simulink model "present1"  (Simulink 7.6)
settings: Solver=ode45  StartTime=0.0  StopTime=10.0  RelTol=1e-3
settings Model: Creator=jordan  LastModifiedBy=jordan

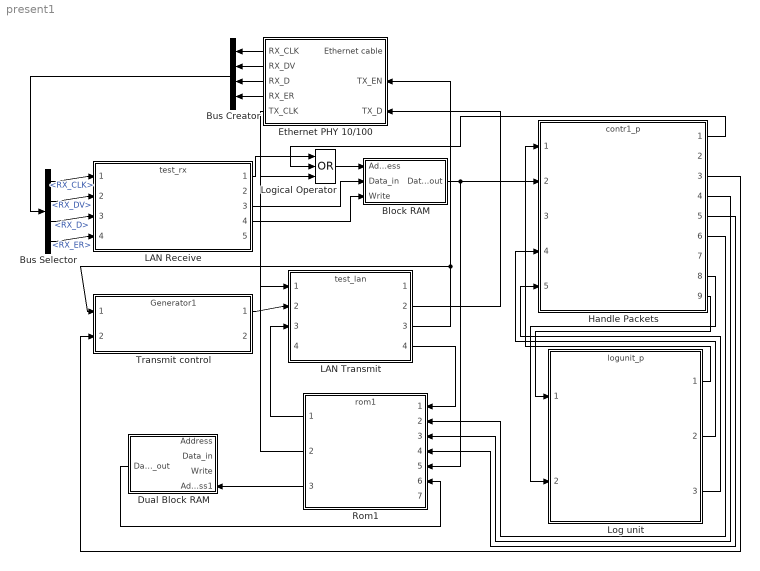
== system present1 ==
  Block RAM : Subsystem
  Bus Creator : BusCreator  Inputs='RX_CLK','RX_DV','RX_D','RX_ER'
  Bus Selector : BusSelector  OutputSignals=RX_CLK,RX_DV,RX_D,RX_ER
  Dual Block RAM : Subsystem
  Ethernet PHY 10/100 : Subsystem
  Handle Packets : ModelReference  ModelNameDialog=contr1_p  SimulationMode=Normal  ModelReferenceVersion=1.463  CopyOfModelName=contr1_p
  LAN Receive : ModelReference  ModelNameDialog=test_rx  SimulationMode=Normal  ModelReferenceVersion=1.280  CopyOfModelName=test_rx
  LAN Transmit : ModelReference  ModelNameDialog=test_lan  SimulationMode=Normal  ModelReferenceVersion=1.197  CopyOfModelName=test_lan
  Log unit : ModelReference  ModelNameDialog=logunit_p  SimulationMode=Normal  ModelReferenceVersion=1.518  CopyOfModelName=logunit_p
  Logical Operator : Logic  Operator=OR  Inputs=3  AllPortsSameDT=off  OutDataTypeStr=boolean
  Rom1 : ModelReference  ModelNameDialog=rom1  SimulationMode=Normal  ModelReferenceVersion=1.162  CopyOfModelName=rom1
  Transmit control : ModelReference  ModelNameDialog=Generator1  SimulationMode=Normal  ModelReferenceVersion=1.103  CopyOfModelName=Generator1
  wires:
  Block RAM/1(Data_out) -> Handle Packets/2, Rom1/5
  LAN Receive/3 -> Block RAM/2(Data_in)
  LAN Receive/4 -> Block RAM/3(Write)
  LAN Receive/1 -> Logical Operator/1
  Transmit control/1 -> LAN Transmit/2
  LAN Transmit/3 -> Transmit control/1, Ethernet PHY 10/100/2(TX_EN)
  Logical Operator/1 -> Block RAM/1(Address)
  Rom1/1 -> LAN Transmit/3
  LAN Transmit/4 -> Rom1/1
  Rom1/2 -> Logical Operator/3
  Ethernet PHY 10/100/1(RX_CLK) -> Bus Creator/1
  Ethernet PHY 10/100/2(RX_DV) -> Bus Creator/2
  Ethernet PHY 10/100/3(RX_D) -> Bus Creator/3
  Ethernet PHY 10/100/4(RX_ER) -> Bus Creator/4
  Bus Selector/1 -> LAN Receive/1  "<RX_CLK>"
  Bus Selector/2 -> LAN Receive/2  "<RX_DV>"
  Bus Selector/3 -> LAN Receive/3  "<RX_D>"
  Bus Selector/4 -> LAN Receive/4  "<RX_ER>"
  LAN Transmit/2 -> Ethernet PHY 10/100/3(TX_D)
  Ethernet PHY 10/100/5(TX_CLK) -> LAN Transmit/1
  Dual Block RAM/1(Data_out) -> Rom1/6
  Rom1/3 -> Dual Block RAM/4(Address1)
  Log unit/1 -> Handle Packets/1
  Bus Creator/1 -> Bus Selector/1
  Log unit/2 -> Handle Packets/4
  Log unit/3 -> Handle Packets/5
  Handle Packets/1 -> Logical Operator/2
  Handle Packets/6 -> Rom1/2
  Handle Packets/4 -> Rom1/3
  Handle Packets/5 -> Rom1/4
  Handle Packets/3 -> Transmit control/2
  Handle Packets/9 -> Log unit/1
  Handle Packets/8 -> Log unit/2

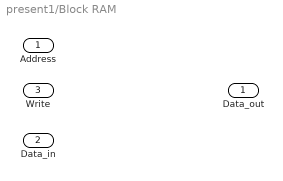
== system present1/Block RAM ==
  Address : Inport  OutDataTypeStr=boolean
  Data_in : Inport  Port=2  OutDataTypeStr=boolean
  Write : Inport  Port=3  OutDataTypeStr=boolean
  Data_out : Outport

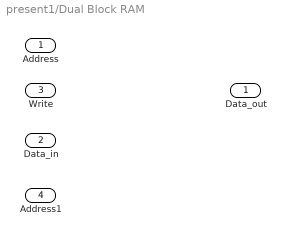
== system present1/Dual Block RAM ==
  Address : Inport  OutDataTypeStr=boolean
  Data_in : Inport  Port=2  OutDataTypeStr=boolean
  Write : Inport  Port=3  OutDataTypeStr=boolean
  Address1 : Inport  Port=4  OutDataTypeStr=boolean
  Data_out : Outport

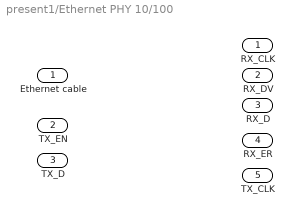
== system present1/Ethernet PHY 10/100 ==
  Ethernet cable : Inport  OutDataTypeStr=boolean
  TX_EN : Inport  Port=2  OutDataTypeStr=boolean
  TX_D : Inport  Port=3  OutDataTypeStr=boolean
  RX_CLK : Outport
  RX_DV : Outport  Port=2
  RX_D : Outport  Port=3
  RX_ER : Outport  Port=4
  TX_CLK : Outport  Port=5
